simulink model "tqdtqr_rebuild_V3"  (R2021b)
settings: Solver=VariableStepAuto  StartTime=0.0  StopTime=10.0  RelTol=1e-3
undefined symbols (not defined in the file): ATQD_AfterTqMinGain_X_Deg, ATQD_APSCreepBaseTqD_X_kph, ATQD_APSCreepBaseTqD_Y_Deg, ATQD_APSCreepBaseTqR_X_kph, ATQD_APSCreepBaseTqR_Y_Deg, ATQD_APSCreepIterm_X_kph, ATQD_APSCreepIterm_Y_kph, ATQD_APSCreepPterm_X_kph, ATQD_APSCreepPterm_Y_kph, ATQD_APSDecReq_X_kph, ATQD_APSDecReq_Y_mps2, ATQD_APSDecReqCMD_X_kph, ATQD_APSDecReqTs_X_pct, ATQD_APSDecTimeGain_X_Deg, ATQD_APSDecTimeGain_Y_s, ATQD_APSReqLowSpd_X_Deg, ATQD_AutoHoldReleaseBPS_X_Deg, ATQD_AWDLoadTrqnsGain_X_kg, ATQD_AWDLoadTrqnsGain_Y_pct, ATQD_BOSEnBPSPosn_X_kph, ATQD_BOSMap_X_rpm, ATQD_BOSMap_Y_pct, ATQD_CreepBaseTqD_X_kph, ATQD_CreepBaseTqD_Y_Deg, ATQD_CreepBaseTqR_X_kph, ATQD_CreepBaseTqR_Y_Deg, ATQD_CreepBPSDisPosn_X_Deg, ATQD_CreepBPSDisPosnR_X_Deg, ATQD_CreepBPSEnPosn_X_Deg, ATQD_CreepBPSEnPosnR_X_Deg, ATQD_CreepDeltaTq_X_kph, ATQD_CreepIterm_X_kph, ATQD_CreepIterm_Y_kph, ATQD_CreepItermMaxLimit_X_pct, ATQD_CreepPreloadTime_X_kph, ATQD_CreepPreloadTq_X_kph, ATQD_CreepPreloadTq_Y_s, ATQD_CreepProtTq_X_Deg, ATQD_CreepPterm_X_kph, ATQD_CreepPterm_Y_kph, ATQD_CreepRrTqSpRat_X_rpm, ATQD_CreepRrTqSpRat_Y_Nm, ATQD_CreepTargetSpdD_X_pct, ATQD_CreepTargetSpdR_X_pct, ATQD_CreepUpLimitTq_X_rpm, ATQD_DecIneOPDHoldEnDelay_X_Deg, ATQD_DecIneOPDHoldEnDelay_Y_bar, ATQD_ECOTqMapD_X_rpm, ATQD_ECOTqMapD_Y_pct, ATQD_EMTqMapD_X_rpm, ATQD_EMTqMapD_Y_pct, ATQD_EOPDTqMapDCon_X_rpm, ATQD_EOPDTqMapDCon_Y_Deg, ATQD_EstInitVehWeight_X_c, ATQD_FAfterTqCMDGain_X_rpm, ATQD_FAfterTqCMDGain_Y_pct, ATQD_ForceLowSpd_X_Deg, ATQD_ForcePLimitSpd_X_Deg, ATQD_FrLossMAPLowV_X_rpm, ATQD_FrLossMAPLowV_Y_Nm ... (+949)
libraries: simulink x235, hcu_lib x208, tqr x63, tqd x6
(part 22 of 37)

== system tqdtqr_rebuild_V3/Input_Convert/Signal function/OPD Hold/OPDHold Request  ==
  VTQD_VehActSpd_kph : Inport
  VTQD_APSStaSys_enum : Inport  Port=2
  VTQD_AutiHoldRelease_flg : Inport  Port=3
  task_time_s : Inport  Port=4
  VVMC_EstSlope_Deg : Inport  Port=5
  VTQD_OPDHoldForceEn_flg : Inport  Port=6
  AND : Logic  AllPortsSameDT=off  OutDataTypeStr=boolean
  AND1 : Logic  Inputs=3  AllPortsSameDT=off  OutDataTypeStr=boolean
  AND2 : Logic  Operator=OR  AllPortsSameDT=off  OutDataTypeStr=boolean
  AND3 : Logic  AllPortsSameDT=off  OutDataTypeStr=boolean
  AND4 : Logic  AllPortsSameDT=off  OutDataTypeStr=boolean
  Constant1 : Constant  Value=KTQD_APSReqUpSpd_kph
  Constant10 : Constant  Value=KTQD_APSReqDownSpd_kph
  Constant11 : Constant  Value=KTQD_OPDHoldLampDelayTime_s
  Constant12 : Constant  Value=KTQD_OPDHoldLampEnSpd_kph  OutDataTypeStr=single
  Constant13 : Constant  Value=KTQD_OPDHoldLampDisSpd_kph  OutDataTypeStr=single
  Constant14 : Constant  Value=KTQD_ForceAPSReqUpSpd_kph
  Constant15 : Constant  Value=KTQD_APSReqDelayTime_s
  Constant16 : Constant  Value=KTQD_OPDHoldAlarm_flg_ovrdflg
  Constant17 : Constant  Value=KTQD_OPDHoldAlarm_flg_ovrdval
  Constant2 : Constant  Value=2  OutDataTypeStr=uint8
  Constant3 : Constant  Value=2  OutDataTypeStr=uint8
  Constant4 : Constant  OutDataTypeStr=uint8
  Constant5 : Constant  Value=2  OutDataTypeStr=uint8
  Constant6 : Constant  Value=0  OutDataTypeStr=uint8
  Constant7 : Constant  OutDataTypeStr=uint8
  Constant8 : Constant  OutDataTypeStr=uint8
  Constant9 : Constant  Value=KTQD_APSReqDelayTime_s
  Equal1 : RelationalOperator  Operator=<  OutDataTypeStr=boolean  RndMeth=Simplest
  Equal2 : RelationalOperator  Operator=~=  OutDataTypeStr=boolean  RndMeth=Simplest
  Equal3 : RelationalOperator  Operator===  OutDataTypeStr=boolean  RndMeth=Simplest
  Equal4 : RelationalOperator  Operator===  OutDataTypeStr=boolean  RndMeth=Simplest
  Equal5 : RelationalOperator  Operator===  OutDataTypeStr=boolean  RndMeth=Simplest
  Equal6 : RelationalOperator  Operator=>  OutDataTypeStr=boolean  RndMeth=Simplest
  MTQD_APSReqLowSpd_Y_kph : Lookup_n-D  NumberOfTableDimensions=1  BreakpointsForDimension1=ATQD_APSReqLowSpd_X_Deg  Table=MTQD_APSReqLowSpd_Y_kph  InternalRulePriority=Speed  RndMeth=Simplest  InputSameDT=on
  MTQD_ForceLowSpd_Y_kph : Lookup_n-D  NumberOfTableDimensions=1  BreakpointsForDimension1=ATQD_ForceLowSpd_X_Deg  Table=MTQD_ForceLowSpd_Y_kph  InternalRulePriority=Speed  RndMeth=Simplest  InputSameDT=on
  NOT1 : Logic  Operator=NOT  AllPortsSameDT=off  OutDataTypeStr=boolean
  NOT2 : Logic  Operator=NOT  AllPortsSameDT=off  OutDataTypeStr=boolean
  Relational Operator1 : RelationalOperator  Operator=<  OutDataTypeStr=boolean  RndMeth=Simplest
  Relational Operator2 : RelationalOperator  OutDataTypeStr=boolean  RndMeth=Simplest
  Relational Operator3 : RelationalOperator  Operator=<  OutDataTypeStr=boolean  RndMeth=Simplest
  Relational Operator4 : RelationalOperator  Operator=>  OutDataTypeStr=boolean  RndMeth=Simplest
  Relational Operator5 : RelationalOperator  OutDataTypeStr=boolean  RndMeth=Simplest
  Relay : Relay  OnSwitchValue=KTQD_OPDHoldGradeUp_Deg  OffSwitchValue=KTQD_OPDHoldGradeDown_Deg  OutDataTypeStr=boolean
      settings: AttributesFormatString=|
      | On: %<OffSwitchValue>
      | Off: %<OnSwitchValue>
  SR_Latch : hcu_lib/Basic_Blocks/SR_Latch
  SR_Latch1 : hcu_lib/Basic_Blocks/SR_Latch
  Switch{,1..5} (6 alike) : Switch  Criteria=u2 ~= 0
      settings: AttributesFormatString=%<Criteria>
  Timer : hcu_lib/Basic_Blocks/Timer
  VTQD_APSReqTimer_s : Outport
  VTQD_APSReq_enum : Outport  Port=2
  VTQD_APSDecReqA_flg : Outport  Port=3
  VTQD_OPDHoldLamp_flg : Outport  Port=4
  VTQD_OPDHoldAlarm_flg : Outport  Port=5
  wires:
  AND3/1 -> [VTQD_OPDHoldLamp_flg]  "VTQD_OPDHoldLamp_flg"
  SR_Latch1/1 -> AND3/2  "VTQD_OPDHoldSpdEnLamp_flg"
  Equal6/1 -> AND3/1
  Relational Operator4/1 -> SR_Latch1/2
  Constant13/1 -> Relational Operator4/2
  [VTQD_VehActSpd_kph] -> Relational Operator4/1
  Constant12/1 -> Relational Operator3/2
  Relational Operator3/1 -> SR_Latch1/1
  [VTQD_VehActSpd_kph] -> Relational Operator3/1
  [VTQD_OPDHoldLamp_flg] -> VTQD_OPDHoldLamp_flg/1
  [VTQD_APSReqTimer_s] -> Equal6/1
  Constant11/1 -> Equal6/2
  Constant10/1 -> Switch/3
  Constant1/1 -> Switch/1
  Relay/1 -> Switch/2  "VTQD_OPDHoldUpDown_flg"
  [VVMC_EstSlope_Deg] -> Relay/1
  Equal2/1 -> AND2/2
  [VTQD_APSStaSys_enum] -> Equal2/1
  Constant3/1 -> Equal2/2
  [VTQD_AutiHoldRelease_flg] -> AND2/1
  AND2/1 -> SR_Latch/2
  Relational Operator1/1 -> SR_Latch/1
  SR_Latch/1 -> AND1/1
  [VVMC_EstSlope_Deg] -> MTQD_APSReqLowSpd_Y_kph/1
  VVMC_EstSlope_Deg/1 -> [VVMC_EstSlope_Deg]
  [VTQD_AutiHoldRelease_flg] -> NOT1/1
  [VTQD_APSDecReqA_flg] -> VTQD_APSDecReqA_flg/1
  [VTQD_APSReq_enum] -> VTQD_APSReq_enum/1
  [VTQD_APSReqTimer_s] -> VTQD_APSReqTimer_s/1
  task_time_s/1 -> [task_time_s]
  VTQD_AutiHoldRelease_flg/1 -> [VTQD_AutiHoldRelease_flg]
  VTQD_APSStaSys_enum/1 -> [VTQD_APSStaSys_enum]
  VTQD_VehActSpd_kph/1 -> [VTQD_VehActSpd_kph]
  Constant5/1 -> Equal4/2
  AND1/1 -> Timer/1, NOT2/1  "VTQD_APSStasysLow_flg"
  [VTQD_VehActSpd_kph] -> Relational Operator1/1
  [VTQD_APSStaSys_enum] -> Equal4/1
  Equal1/1 -> AND/1
  Switch1/1 -> Switch2/3
  Constant2/1 -> Equal3/2
  [VTQD_APSReq_enum] -> Equal5/1
  Constant7/1 -> Equal5/2
  NOT1/1 -> AND1/3
  [VTQD_APSReqUpSpd_kph] -> Equal1/2
  Equal5/1 -> [VTQD_APSDecReqA_flg]  "VTQD_APSDecReqA_flg"
  [VTQD_VehActSpd_kph] -> Equal1/1
  [VTQD_APSStaSys_enum] -> Equal3/1
  Equal4/1 -> AND1/2
  Constant8/1 -> Switch2/1
  Relational Operator2/1 -> Switch2/2
  Timer/1 -> Relational Operator2/1, [VTQD_APSReqTimer_s]  "VTQD_APSReqTimer_s"
  Constant6/1 -> Switch1/3
  Equal3/1 -> AND/2
  Constant9/1 -> Timer/4, Relational Operator2/2
  AND/1 -> Switch1/2  "VTQD_APSStasysUp_flg"
  Switch2/1 -> [VTQD_APSReq_enum]  "VTQD_APSReq_enum"
  NOT2/1 -> Timer/2
  Constant4/1 -> Switch1/1
  [task_time_s] -> Timer/3
  Constant14/1 -> Switch4/1
  [VTQD_OPDHoldForceEn_flg] -> Switch4/2
  Switch/1 -> Switch4/3
  Switch4/1 -> [VTQD_APSReqUpSpd_kph]  "VTQD_APSReqUpSpd_kph"
  [VVMC_EstSlope_Deg] -> MTQD_ForceLowSpd_Y_kph/1
  MTQD_ForceLowSpd_Y_kph/1 -> Switch3/1  "VTQD_ForceReqLowSpd_kph"
  Switch3/1 -> [VTQD_OPDHoldReqLowSpd_kph]  "VTQD_OPDHoldReqLowSpd_kph"
  [VTQD_OPDHoldForceEn_flg] -> Switch3/2
  MTQD_APSReqLowSpd_Y_kph/1 -> Switch3/3  "VTQD_APSReqLowSpd_kph"
  [VTQD_OPDHoldReqLowSpd_kph] -> Relational Operator1/2
  Constant15/1 -> Relational Operator5/2
  AND4/1 -> Switch5/3
  Constant16/1 -> Switch5/2
  [VTQD_APSReqTimer_s] -> Relational Operator5/1
  Switch5/1 -> [VTQD_OPDHoldAlarm_flg]  "VTQD_OPDHoldAlarm_flg"
  Constant17/1 -> Switch5/1
  Relational Operator5/1 -> AND4/1
  [VTQD_OPDHoldForceEn_flg] -> AND4/2
  VTQD_OPDHoldForceEn_flg/1 -> [VTQD_OPDHoldForceEn_flg]
  [VTQD_OPDHoldAlarm_flg] -> VTQD_OPDHoldAlarm_flg/1

== system tqdtqr_rebuild_V3/Input_Convert/Signal function/OPD Hold/Parking Requeest Backup ==
  note: Park request
  note: Allow park
  VTQD_APSReq_enum : Inport
  VTQD_APSReqTimer_s : Inport  Port=2
  VTQD_ParkRequest_flg : Inport  Port=3
  task_time_s : Inport  Port=4
  VTQD_AutiHoldRelease_flg : Inport  Port=5
  AND : Logic  AllPortsSameDT=off  OutDataTypeStr=boolean
  AND1 : Logic  AllPortsSameDT=off  OutDataTypeStr=boolean
  AND3 : Logic  Inputs=3  AllPortsSameDT=off  OutDataTypeStr=boolean
  Constant1 : Constant  Value=KTQD_APSReqDelayTime_s
  Constant16 : Constant  OutDataTypeStr=uint8
  Constant17 : Constant  Value=TRUE  OutDataTypeStr=uint8
  Constant2 : Constant  Value=KTQD_APSReqDelayTime_s
  Constant3 : Constant  Value=KTQD_OPDHoldBrkSW_flg
  Constant4 : Constant  Value=KTQD_OPDHoldAllowPark_flg
  Constant5 : Constant  Value=KTQD_OPDHoldAllowPark_s
  Constant6 : Constant  Value=KTQD_OPDHoldAllowGearPSW_flg
  DelayEnable : hcu_lib/Basic_Blocks/DelayEnable
  Equal6 : RelationalOperator  Operator===  OutDataTypeStr=boolean  RndMeth=Simplest
  NOT : Logic  Operator=NOT  AllPortsSameDT=off  OutDataTypeStr=boolean
  OR : Logic  Operator=OR  AllPortsSameDT=off  OutDataTypeStr=boolean
  Relational Operator1 : RelationalOperator  OutDataTypeStr=boolean  RndMeth=Simplest
  Relational Operator6 : RelationalOperator  OutDataTypeStr=boolean  RndMeth=Simplest
  SR_Latch : hcu_lib/Basic_Blocks/SR_Latch
  Switch4 : Switch  Criteria=u2 ~= 0
      settings: AttributesFormatString=%<Criteria>
  VTQD_ActParkRequest_flg : Outport
  VTQD_OPDHoldAllowPark_flg : Outport  Port=2
  wires:
  [VTQD_OPDHoldAllowPark_flg] -> VTQD_OPDHoldAllowPark_flg/1
  Constant6/1 -> NOT/1
  NOT/1 -> AND1/2
  AND1/1 -> OR/2
  [VTQD_OPDHoldAllowPark_flg] -> AND1/1
  [task_time_s] -> DelayEnable/3
  AND3/1 -> OR/1
  OR/1 -> Switch4/2
  SR_Latch/1 -> [VTQD_OPDHoldAllowPark_flg]  "VTQD_OPDHoldAllowPark_flg"
  VTQD_AutiHoldRelease_flg/1 -> [VTQD_AutiHoldRelease_flg]
  [VTQD_AutiHoldRelease_flg] -> SR_Latch/2
  DelayEnable/1 -> SR_Latch/1
  Constant5/1 -> DelayEnable/2
  Constant4/1 -> AND/2
  Relational Operator1/1 -> AND/1
  AND/1 -> DelayEnable/1
  task_time_s/1 -> [task_time_s]
  [VTQD_APSReqTimer_s] -> Relational Operator1/1
  Constant2/1 -> Relational Operator1/2
  [VTQD_ActParkRequest_flg] -> VTQD_ActParkRequest_flg/1
  VTQD_ParkRequest_flg/1 -> [VTQD_ParkRequest_flg]
  VTQD_APSReqTimer_s/1 -> [VTQD_APSReqTimer_s]
  VTQD_APSReq_enum/1 -> [VTQD_APSReq_enum]
  [VTQD_APSReqTimer_s] -> Relational Operator6/1
  Switch4/1 -> [VTQD_ActParkRequest_flg]  "VTQD_ActParkRequest_flg"
  Constant16/1 -> Equal6/2
  Constant17/1 -> Switch4/1
  [VTQD_ParkRequest_flg] -> Switch4/3
  Relational Operator6/1 -> AND3/3
  [VTQD_APSReq_enum] -> Equal6/1
  Equal6/1 -> AND3/1
  Constant1/1 -> Relational Operator6/2
  Constant3/1 -> AND3/2

== system tqdtqr_rebuild_V3/Input_Convert/Signal function/OPD Hold/Release Condition ==
  note: Release auto hold
  note: OPD release in reverse condition
  note: OPD Enable Flag
  note: Calculate Tq to release OPD disable
  note: Calulaye Tq to release OPD enable
  note: OPD detect time
  VVMC_EstSlope_Deg : Inport
  VTQD_VehActSpd_kph : Inport  Port=2
  VTQR_NoABSFEDUWhlTqReq_Nm : Inport  Port=3
  VTQR_NoABSREDUWhlTqReq_Nm : Inport  Port=4
  VTQD_ActBPSPosn_pct : Inport  Port=5
  task_time_s : Inport  Port=6
  VTQD_APSReqTimer_s : Inport  Port=7
  VTQD_LowIdleAccPedal_flg : Inport  Port=8
  VTQD_OPDHoldRgnOn2Off_flg : Inport  Port=9
  AND : Logic  Inputs=3  AllPortsSameDT=off  OutDataTypeStr=boolean
  AND1 : Logic  AllPortsSameDT=off  OutDataTypeStr=boolean
  AND2 : Logic  AllPortsSameDT=off  OutDataTypeStr=boolean
  AND3 : Logic  AllPortsSameDT=off  OutDataTypeStr=boolean
  Add : Sum
  Add1 : Sum  Inputs=+-+
  Add6 : Sum
  Add7 : Sum
  Constant1 : Constant  Value=KTQD_APSRelDisTqDev_Nm
  Constant{5,10,23,30} (4 alike) : Constant  Value=ZERO_FLOAT
  Constant2 : Constant  Value=KTQD_OPDHoldDownEnTime_s
  Constant36 : Constant  Value=KTQD_OPDHoldRelDetSpd_kph
  Constant4 : Constant  Value=KTQD_OPDHoldRelTqGain_Nm
  Constant6 : Constant  Value=KTQD_OPDHoldDetRevSpd_kph
  Constant7 : Constant  Value=KTQD_OPDHoldLiftRevSpd_kph
  Constant8 : Constant  Value=KTQD_APSDecReqMaxTime_s
  Constant9 : Constant  Value=KTQD_OPDHoldRelTqGain_Nm
  Delay{,1..2,4..7} (7 alike) : Delay  DelayLength=1  InitialCondition=single(0)
      settings: AttributesFormatString=%<InitialCondition>
  Delay3 : Delay  DelayLength=1
  DelayEnable : hcu_lib/Basic_Blocks/DelayEnable
  DelayEnable1 : hcu_lib/Basic_Blocks/DelayEnable
  Detect Increase : simulink/Logic and Bit Operations/Detect Increase  vinit=0.0  OutDataTypeStr=boolean
  Detect Increase1 : simulink/Logic and Bit Operations/Detect Increase  vinit=0.0  OutDataTypeStr=boolean
  Detect Increase2 : simulink/Logic and Bit Operations/Detect Increase  vinit=0.0  OutDataTypeStr=boolean
  MTQD_AutoHoldReleaseBPS_Y_pct : Lookup_n-D  NumberOfTableDimensions=1  BreakpointsForDimension1=ATQD_AutoHoldReleaseBPS_X_Deg  Table=MTQD_AutoHoldReleaseBPS_Y_pct  InternalRulePriority=Speed  RndMeth=Simplest  InputSameDT=on
  MTQD_OPDHoldDownRelDelay_Y_s : Lookup_n-D  NumberOfTableDimensions=1  BreakpointsForDimension1=ATQD_OPDHoldDownRelDelay_X_Deg  Table=MTQD_OPDHoldDownRelDelay_Y_s  InternalRulePriority=Speed  RndMeth=Simplest  InputSameDT=on
  MTQD_OPDHoldRelDetTime_Y_s : Lookup_n-D  NumberOfTableDimensions=1  BreakpointsForDimension1=ATQD_OPDHoldRelDetTime_X_Deg  Table=MTQD_OPDHoldRelDetTime_Y_s  InternalRulePriority=Speed  RndMeth=Simplest  InputSameDT=on
  MTQD_OPDHoldReleaseTq_Y_Nm{,1..3} (4 alike) : Lookup_n-D  NumberOfTableDimensions=1  BreakpointsForDimension1=ATQD_OPDHoldReleaseTq_X_Deg  Table=MTQD_OPDHoldReleaseTq_Y_Nm  InternalRulePriority=Speed  RndMeth=Simplest  InputSameDT=on
  Max : MinMax  Function=max  Inputs=2
  Max1 : MinMax  Function=max  Inputs=2
  Max2 : MinMax  Function=max  Inputs=2
  NOT{,1..5} (6 alike) : Logic  Operator=NOT  AllPortsSameDT=off  OutDataTypeStr=boolean
  OR : Logic  Operator=OR  AllPortsSameDT=off  OutDataTypeStr=boolean
  OR1 : Logic  Operator=OR  AllPortsSameDT=off  OutDataTypeStr=boolean
  OR2 : Logic  Operator=OR  AllPortsSameDT=off  OutDataTypeStr=boolean
  OR3 : Logic  Operator=OR  Inputs=3  AllPortsSameDT=off  OutDataTypeStr=boolean
  Relational Operator : RelationalOperator  Operator=>  OutDataTypeStr=boolean  RndMeth=Simplest
  Relational Operator1 : RelationalOperator  Operator=<=  OutDataTypeStr=boolean  RndMeth=Simplest
  Relational Operator3 : RelationalOperator  Operator=<=  OutDataTypeStr=boolean  RndMeth=Simplest
  Relational Operator4 : RelationalOperator  OutDataTypeStr=boolean  RndMeth=Simplest
  Relational Operator5 : RelationalOperator  Operator=<  OutDataTypeStr=boolean  RndMeth=Simplest
  Relational Operator6 : RelationalOperator  Operator=>  OutDataTypeStr=boolean  RndMeth=Simplest
  Relational Operator7 : RelationalOperator  OutDataTypeStr=boolean  RndMeth=Simplest
  Relational Operator9 : RelationalOperator  OutDataTypeStr=boolean  RndMeth=Simplest
  Relay : Relay  OnSwitchValue=KTQD_OPDHoldGradeUp_Deg  OffSwitchValue=KTQD_OPDHoldGradeDown_Deg  OutDataTypeStr=boolean
      settings: AttributesFormatString=|
      | Off: %<OffSwitchValue>
      | On: %<OnSwitchValue>
  Relay1 : Relay  OnSwitchValue=KTQD_OPDHoldGradeUp_Deg  OffSwitchValue=KTQD_OPDHoldGradeDown_Deg  OutDataTypeStr=boolean
      settings: AttributesFormatString=|
      | Off: %<OffSwitchValue>
      | On: %<OnSwitchValue>
  SR_Latch : hcu_lib/Basic_Blocks/SR_Latch
  SR_Latch1 : hcu_lib/Basic_Blocks/SR_Latch
  Switch{,1..6} (7 alike) : Switch  Criteria=u2 ~= 0
      settings: AttributesFormatString=%<Criteria>
  VTQD_AutoHoldRelease_flg : Outport
  VTQD_OPDHoldEnRel_flg : Outport  Port=2
  VTQD_OPDHoldActRelTq_Nm : Outport  Port=3
  wires:
  [VTQD_OPDHoldActRelTq_Nm] -> VTQD_OPDHoldActRelTq_Nm/1
  OR3/1 -> SR_Latch1/2
  [VVMC_EstSlope_Deg] -> MTQD_OPDHoldReleaseTq_Y_Nm2/1
  Max/1 -> Switch4/1
  Relational Operator6/1 -> OR3/2
  NOT1/1 -> OR1/2
  Constant1/1 -> Add1/2
  [VTQD_OPDHoldEnRel_flg] -> AND2/1
  [VTQD_VehActSpd_kph] -> Relational Operator6/1
  NOT2/1 -> AND1/1
  Switch/1 -> OR/2
  Constant9/1 -> Switch3/1
  AND3/1 -> OR3/3
  Constant5/1 -> Switch2/3
  Switch4/1 -> Add1/3, Delay2/1
  Constant7/1 -> Relational Operator6/2
  Relational Operator7/1 -> AND3/2
  Delay1/1 -> Relational Operator7/1
  MTQD_OPDHoldReleaseTq_Y_Nm3/1 -> Max2/2
  [VVMC_EstSlope_Deg] -> MTQD_OPDHoldReleaseTq_Y_Nm1/1
  Switch3/1 -> Add1/1
  [VTQD_OPDHoldRelReverse_flg] -> Switch2/2
  Add6/1 -> Relational Operator4/1  "VTQD_OPDHoldEnRelTq_Nm"
  [VTQD_LowIdleAccPedal_flg] -> Detect Increase/1
  MTQD_OPDHoldReleaseTq_Y_Nm2/1 -> Max/2
  Constant10/1 -> Switch3/3
  [VTQD_APSReqTimer_s] -> Delay1/1
  NOT4/1 -> DelayEnable1/1
  Constant36/1 -> Relational Operator9/2
  [VTQD_LowIdleAccPedal_flg] -> NOT5/1
  [VTQD_LowIdleAccPedal_flg] -> AND3/1
  AND1/1 -> Switch/1
  [VTQD_OPDHoldEnRel_flg] -> AND1/2
  Delay2/1 -> Max/1
  [VTQD_VehActSpd_kph] -> Relational Operator3/1
  OR2/1 -> SR_Latch/2
  Constant8/1 -> Relational Operator7/2
  Delay/1 -> Relational Operator1/1
  [VTQD_OPDHoldRelReverse_flg] -> Switch4/2
  Add/1 -> [VTQD_OPDHoldActRelTq_Nm]  "VTQD_OPDHoldActRelTq_Nm"
  Relay/1 -> NOT/1
  MTQD_OPDHoldReleaseTq_Y_Nm1/1 -> Switch4/3
  NOT5/1 -> AND2/2
  Switch2/1 -> Add/1
  [VTQD_OPDHoldRelReverse_flg] -> Switch3/2
  MTQD_OPDHoldRelDetTime_Y_s/1 -> Switch5/3
  [VTQD_LowIdleAccPedal_flg] -> NOT4/1
  Constant23/1 -> Max1/2
  [VTQD_OPDHoldRelReverse_flg] -> Switch6/2
  [VTQD_OPDHoldRelReverse_flg] -> Detect Increase2/1
  NOT3/1 -> Switch1/2
  [VTQD_APSReqTimer_s] -> Delay/1
  [VVMC_EstSlope_Deg] -> MTQD_OPDHoldReleaseTq_Y_Nm3/1
  Switch6/1 -> Delay3/1, Add/2  "VTQD_OPDHoldReleaseTq_Nm"
  Add7/1 -> Relational Operator5/1  "VTQD_OPDHoldDisRelTq_Nm"
  Detect Increase/1 -> OR3/1
  Constant6/1 -> Relational Operator3/2
  Max2/1 -> Switch6/1
  Delay3/1 -> Max2/1
  [VTQD_OPDHoldDownRelDelay_s] -> DelayEnable1/2
  Relational Operator3/1 -> Detect Increase1/1
  MTQD_OPDHoldReleaseTq_Y_Nm/1 -> Switch6/3
  OR/1 -> [VTQD_AutoHoldRelease_flg]  "VTQD_AutoHoldRelease_flg"
  MTQD_AutoHoldReleaseBPS_Y_pct/1 -> Relational Operator/2  "VTQD_AutoHoldReleaseAPS_pct"
  Switch5/1 -> [VTQD_OPDHoldRelDetTime_s]  "VTQD_OPDHoldRelDetTime_s"
  [VVMC_EstSlope_Deg] -> MTQD_OPDHoldRelDetTime_Y_s/1
  [VVMC_EstSlope_Deg] -> MTQD_AutoHoldReleaseBPS_Y_pct/1
  Relational Operator9/1 -> Switch5/2
  [VTQD_VehActSpd_kph] -> Relational Operator9/1
  Max1/1 -> Relational Operator5/2
  [VTQR_NoABSREDUWhlTqReq_Nm] -> Delay7/1
  DelayEnable/1 -> [VTQD_OPDHoldEnRel_flg]  "VTQD_OPDHoldEnRel_flg"
  [VVMC_EstSlope_Deg] -> MTQD_OPDHoldReleaseTq_Y_Nm/1
  Add1/1 -> Max1/1
  [VTQD_ActBPSPosn_pct] -> Relational Operator/1
  [task_time_s] -> DelayEnable/3
  [VTQR_NoABSREDUWhlTqReq_Nm] -> Delay5/1
  [VTQR_NoABSFEDUWhlTqReq_Nm] -> Delay4/1
  [VVMC_EstSlope_Deg] -> Relay/1
  AND/1 -> OR/1
  [VTQD_OPDHoldRelDetTime_s] -> DelayEnable/2
  Relational Operator1/1 -> AND/1
  Relational Operator/1 -> OR1/1
  [VTQD_OPDHoldRgnOn2Off_flg] -> Switch/2
  [VTQD_LowIdleAccPedal_flg] -> NOT1/1
  AND2/1 -> Switch1/3
  Switch1/1 -> Switch/3
  OR1/1 -> AND/3
  Constant2/1 -> Relational Operator1/2
  Relay1/1 -> NOT3/1
  [VVMC_EstSlope_Deg] -> Relay1/1
  NOT/1 -> AND/2
  Constant30/1 -> Switch5/1
  [VTQD_LowIdleAccPedal_flg] -> NOT2/1
  [task_time_s] -> DelayEnable1/3
  [VVMC_EstSlope_Deg] -> MTQD_OPDHoldDownRelDelay_Y_s/1
  Constant4/1 -> Switch2/1
  MTQD_OPDHoldDownRelDelay_Y_s/1 -> [VTQD_OPDHoldDownRelDelay_s]  "VTQD_OPDHoldDownRelDelay_s"
  SR_Latch1/1 -> [VTQD_OPDHoldRelReverse_flg]  "VTQD_OPDHoldRelReverse_flg"
  DelayEnable1/1 -> Switch1/1
  Detect Increase1/1 -> SR_Latch1/1
  Detect Increase2/1 -> OR2/1
  SR_Latch/1 -> DelayEnable/1  "VTQD_OPDHoldEnRelLatch_flg"
  VTQD_OPDHoldRgnOn2Off_flg/1 -> [VTQD_OPDHoldRgnOn2Off_flg]
  VTQD_LowIdleAccPedal_flg/1 -> [VTQD_LowIdleAccPedal_flg]
  VTQD_APSReqTimer_s/1 -> [VTQD_APSReqTimer_s]
  [VTQD_OPDHoldEnRel_flg] -> VTQD_OPDHoldEnRel_flg/1
  [VTQD_AutoHoldRelease_flg] -> VTQD_AutoHoldRelease_flg/1
  task_time_s/1 -> [task_time_s]
  VTQD_ActBPSPosn_pct/1 -> [VTQD_ActBPSPosn_pct]
  VTQR_NoABSREDUWhlTqReq_Nm/1 -> [VTQR_NoABSREDUWhlTqReq_Nm]
  VTQR_NoABSFEDUWhlTqReq_Nm/1 -> [VTQR_NoABSFEDUWhlTqReq_Nm]
  VTQD_VehActSpd_kph/1 -> [VTQD_VehActSpd_kph]
  VVMC_EstSlope_Deg/1 -> [VVMC_EstSlope_Deg]
  Relational Operator4/1 -> [VTQD_OPDHoldEnRelease_flg]  "VTQD_OPDHoldEnRelease_flg"
  [VTQD_OPDHoldEnRelease_flg] -> SR_Latch/1
  [VTQD_OPDHoldActRelTq_Nm] -> Relational Operator4/2
  Relational Operator5/1 -> [VTQD_OPDHoldDisRelease_flg]  "VTQD_OPDHoldDisRelease_flg"
  [VTQD_OPDHoldDisRelease_flg] -> OR2/2
  Delay4/1 -> Add6/1
  Delay5/1 -> Add6/2
  Delay6/1 -> Add7/1
  [VTQR_NoABSFEDUWhlTqReq_Nm] -> Delay6/1
  Delay7/1 -> Add7/2

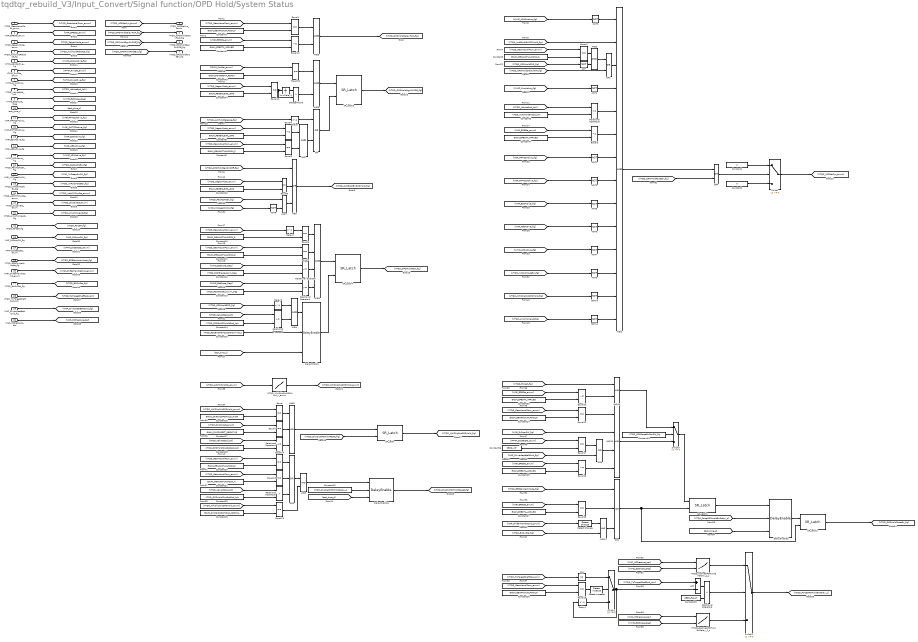
== system tqdtqr_rebuild_V3/Input_Convert/Signal function/OPD Hold/System Status ==
  VTQD_GearActualPosn_enum : Inport
  VINP_EPBSta_enum : Inport  Port=2
  VTQD_RegenMode_enum : Inport  Port=3
  VTQD_AutiHoldRelease_flg : Inport  Port=4
  VVMC_ADASActive_flg : Inport  Port=5
  VPMM_PwrSta_enum : Inport  Port=6
  VVMC_CruzActive_flg : Inport  Port=7
  VTQD_VehActSpd_kph : Inport  Port=8
  VVMC_EstSlope_Deg : Inport  Port=9
  task_time_s : Inport  Port=10
  VINP_FrPTCSActive_flg : Inport  Port=11
  VINP_RrPTCSActive_flg : Inport  Port=12
  VINP_ESCActive_flg : Inport  Port=13
  VINP_ABSActive_flg : Inport  Port=14
  VVMC_APSActive_flg : Inport  Port=15
  VTQD_PedAccTqEn_flg : Inport  Port=16
  VINP_IVICreepOnSW_flg : Inport  Port=17
  VTQD_IVIRockModeEn_flg : Inport  Port=18
  VTQD_ActWhlSkipSta_enum : Inport  Port=19
  VTQD_SkipDirect_enum : Inport  Port=20
  VTQD_LimpHomeAct_flg : Inport  Port=21
  VTQD_ForceP_flg : Inport  Port=22
  VINP_DrDoorSW_flg : Inport  Port=23
  VPMM_DrSeatSta_enum : Inport  Port=24
  VTQD_EPBCarWashMode_flg : Inport  Port=25
  VINP_ShifterHandleCmd_enum : Inport  Port=26
  VTQD_BrkSwSta_flg : Inport  Port=27
  VTQD_TqTargetShaftSpd_rpm : Inport  Port=28
  VINP_DriverSeatBeltCmd_flg : Inport  Port=29
  VINP_MCPressure_bar : Inport  Port=30
  AND{,3..7,9..11} (9 alike) : Logic  AllPortsSameDT=off  OutDataTypeStr=boolean
  AND1 : Logic  Inputs=4  AllPortsSameDT=off  OutDataTypeStr=boolean
  AND12 : Logic  Inputs=4  AllPortsSameDT=off  OutDataTypeStr=boolean
  AND2 : Logic  Inputs=14  AllPortsSameDT=off  OutDataTypeStr=boolean
  AND8 : Logic  Inputs=3  AllPortsSameDT=off  OutDataTypeStr=boolean
  Abs : Abs
  Add : Sum  Inputs=+-
  Constant1 : Constant  Value=2  OutDataTypeStr=uint8
  Constant10 : Constant  Value=ENUM_GEARACTUALPOSN_R
  Constant11 : Constant  Value=ENUM_GEARACTUALPOSN_D
  Constant12 : Constant  Value=KTQD_R2DGradeUpLim_Deg
  Constant13 : Constant  Value=KTQD_R2DGradeLowLim_Deg
  Constant14 : Constant  Value=KTQD_R2DEnOPDHoldSpd_kph
  Constant15 : Constant  Value=KTQD_R2DEnOPDHSpdDelayTime_s
  Constant16 : Constant  Value=ENUM_SKIPDISOPDHOLD_HIGH
  Constant17 : Constant  Value=ENUM_SKIPDIRECT_NEGATIVE
  Constant18 : Constant  Value=KTQD_OPDHoldSkipDetSpd_kph
  Constant19 : Constant  Value=ENUM_SKIPDISOPDHOLD_NORMAL
  Constant2 : Constant  Value=0  OutDataTypeStr=uint8
  Constant{4,9,20,24,28} (5 alike) : Constant  Value=ENUM_GEARACTUALPOSN_P
  Constant21 : Constant  Value=ENUM_GEARACTUALPOSN_N
  Constant22 : Constant  Value=KTQD_SkipRecOPDHoldDelay_s
  Constant23 : Constant  Value=KTQD_OPDHoldSkipDetSpd_kph
  Constant{3,7,25,27,30} (5 alike) : Constant  Value=ENUM_EPBSTA_APPLIED
  Constant26 : Constant  Value=ZERO_INT
  Constant29 : Constant  Value=ZERO_FLOAT
  Constant31 : Constant  Value=KTQD_OPDForceEnConSW_flg
  Constant40 : Constant  Value=ENUM_REGENLEVEL_OPD
  Constant44 : Constant  Value=ENUM_REGENLEVEL_OPD
  Constant45 : Constant  Value=ENUM_POWERSTA_READY
  Constant5 : Constant  Value=ENUM_GEARACTUALPOSN_D
  Constant6 : Constant  Value=KTQD_AutoHoldEnSpd_kph
  Constant8 : Constant  Value=ENUM_REGENLEVEL_OPD
  Delay : Delay  DelayLength=1  InitialCondition=boolean(0)
      settings: AttributesFormatString=%<InitialCondition>
  Delay1 : Delay  DelayLength=1  InitialCondition=single(0)
      settings: AttributesFormatString=%<InitialCondition>
  Delay2 : Delay  DelayLength=1  InitialCondition=uint8(0)
      settings: AttributesFormatString=%<InitialCondition>
  Delay3 : Delay  DelayLength=1  InitialCondition=boolean(0)
      settings: AttributesFormatString=%<InitialCondition>
  DelayEnable : hcu_lib/Basic_Blocks/DelayEnable
  DelayEnable1 : hcu_lib/Basic_Blocks/DelayEnable
  DelayEnable2 : hcu_lib/Basic_Blocks/DelayEnable
  Detect Change : simulink/Logic and Bit Operations/Detect Change  vinit=boolean(0)  OutDataTypeStr=boolean
  Detect Increase : simulink/Logic and Bit Operations/Detect Increase  vinit=boolean(0)  OutDataTypeStr=boolean
  Equal{,1..2,5..9,11..15,17..19,30} (17 alike) : RelationalOperator  Operator===  OutDataTypeStr=boolean  RndMeth=Simplest
  Equal{3..4,10,16,20} (5 alike) : RelationalOperator  Operator=~=  OutDataTypeStr=boolean  RndMeth=Simplest
  GreaterThan3 : RelationalOperator  Operator=>  OutDataTypeStr=boolean  RndMeth=Simplest
  MTQD_AccIneOPDHoldEnDelay_Z_s : Lookup_n-D  BreakpointsForDimension1=ATQD_DecIneOPDHoldEnDelay_Y_bar  BreakpointsForDimension2=ATQD_DecIneOPDHoldEnDelay_X_Deg  Table=MTQD_AccIneOPDHoldEnDelay_Z_s  ExtrapMethod=Clip  InternalRulePriority=Speed  RndMeth=Simplest  InputSameDT=on
      settings: InputPortMap=u0,u1
  MTQD_DecIneOPDHoldEnDelay_Z_s : Lookup_n-D  BreakpointsForDimension1=ATQD_DecIneOPDHoldEnDelay_Y_bar  BreakpointsForDimension2=ATQD_DecIneOPDHoldEnDelay_X_Deg  Table=MTQD_DecIneOPDHoldEnDelay_Z_s  ExtrapMethod=Clip  InternalRulePriority=Speed  RndMeth=Simplest  InputSameDT=on
      settings: InputPortMap=u0,u1
  MTQD_WhlSkipDisOPDHold_Y_enum : Lookup_n-D  NumberOfTableDimensions=1  BreakpointsForDimension1=ATQD_WhlSkipDisOPDHold_X_enum  BreakpointsForDimension1DataTypeStr=uint8  Table=MTQD_WhlSkipDisOPDHold_Y_enum  TableDataTypeStr=uint8  IntermediateResultsDataTypeStr=uint8  ExtrapMethod=Clip  UseLastTableValue=on  InternalRulePriority=Speed  OutDataTypeStr=uint8  RndMeth=Simplest  InputSameDT=on
  NOT{,1..11} (12 alike) : Logic  Operator=NOT  AllPortsSameDT=off  OutDataTypeStr=boolean
  OR{,1,4,6} (4 alike) : Logic  Operator=OR  AllPortsSameDT=off  OutDataTypeStr=boolean
  OR2 : Logic  Operator=OR  Inputs=3  AllPortsSameDT=off  OutDataTypeStr=boolean
  OR3 : Logic  Operator=OR  Inputs=3  AllPortsSameDT=off  OutDataTypeStr=boolean
  OR5 : Logic  Operator=OR  Inputs=3  AllPortsSameDT=off  OutDataTypeStr=boolean
  Relational Operator : RelationalOperator  Operator=<=  OutDataTypeStr=boolean  RndMeth=Simplest
  Relational Operator1 : RelationalOperator  OutDataTypeStr=boolean  RndMeth=Simplest
  Relational Operator2 : RelationalOperator  OutDataTypeStr=boolean  RndMeth=Simplest
  Relational Operator3 : RelationalOperator  Operator=<=  OutDataTypeStr=boolean  RndMeth=Simplest
  Relational Operator4 : RelationalOperator  Operator=<=  OutDataTypeStr=boolean  RndMeth=Simplest
  Relational Operator5 : RelationalOperator  Operator=>  OutDataTypeStr=boolean  RndMeth=Simplest
  Relational Operator6 : RelationalOperator  Operator=<  OutDataTypeStr=boolean  RndMeth=Simplest
  SR_Latch{,1..4} (5 alike) : hcu_lib/Basic_Blocks/SR_Latch
  Switch{,1..3} (4 alike) : Switch  Criteria=u2 ~= 0
      settings: AttributesFormatString=%<Criteria>
  Unit Delay1 : UnitDelay  InitialCondition=boolean(0)  SampleTime=-1  HasFrameUpgradeWarning=on
      settings: AttributesFormatString=%<InitialCondition>
  VTQD_APSStaSys_enum : Outport
  VTQD_OPDHoldDelayForP_flg : Outport  Port=2
  VTQD_OPDHoldRgnOn2Off_flg : Outport  Port=3
  VTQD_OPDHoldForceEn_flg : Outport  Port=4
  wires:
  VTQD_LimpHomeAct_flg/1 -> [VTQD_LimpHomeAct_flg]
  NOT11/1 -> AND2/14
  [VTQD_LimpHomeAct_flg] -> NOT11/1
  NOT10/1 -> AND2/13
  [VTQD_WhlSkipDisOPDHold_flg] -> NOT10/1
  SR_Latch/1 -> [VTQD_WhlSkipDisOPDHold_flg]  "VTQD_WhlSkipDisOPDHold_flg"
  [VTQD_SkipDisOPDHoldReset_flg] -> SR_Latch/2
  DelayEnable1/1 -> [VTQD_SkipDisOPDHoldReset_flg]  "VTQD_SkipDisOPDHoldReset_flg"
  AND9/1 -> DelayEnable1/1
  Equal13/1 -> AND9/2
  OR3/1 -> AND9/1
  Relational Operator5/1 -> OR3/3
  [VTQD_VehActSpd_kph] -> Relational Operator5/1
  Constant23/1 -> Relational Operator5/2
  Constant18/1 -> Relational Operator4/2
  [VTQD_VehActSpd_kph] -> Relational Operator4/1
  Relational Operator4/1 -> AND8/3
  Constant22/1 -> DelayEnable1/2
  [task_time_s] -> DelayEnable1/3
  Equal15/1 -> OR3/2
  Equal14/1 -> OR3/1
  Constant20/1 -> Equal14/2
  Constant21/1 -> Equal15/2
  [VTQD_GearActualPosn_enum] -> Equal15/1
  [VTQD_GearActualPosn_enum] -> Equal14/1
  [VTQD_WhlSkipDisOPDHold_enum] -> Equal13/1
  Constant19/1 -> Equal13/2
  AND8/1 -> SR_Latch/1
  Equal7/1 -> AND8/2
  Equal/1 -> AND8/1
  [VTQD_SkipDirect_enum] -> Equal7/1
  Constant17/1 -> Equal7/2
  Constant16/1 -> Equal/2
  [VTQD_WhlSkipDisOPDHold_enum] -> Equal/1
  MTQD_WhlSkipDisOPDHold_Y_enum/1 -> [VTQD_WhlSkipDisOPDHold_enum]  "VTQD_WhlSkipDisOPDHold_enum"
  [VTQD_ActWhlSkipSta_enum] -> MTQD_WhlSkipDisOPDHold_Y_enum/1
  VTQD_ActWhlSkipSta_enum/1 -> [VTQD_ActWhlSkipSta_enum]
  VTQD_SkipDirect_enum/1 -> [VTQD_SkipDirect_enum]
  NOT1/1 -> AND2/7
  NOT2/1 -> AND2/8
  NOT9/1 -> AND2/12
  [VTQD_IVIRockModeEn_flg] -> NOT9/1
  VTQD_IVIRockModeEn_flg/1 -> [VTQD_IVIRockModeEn_flg]
  VTQD_PedAccTqEn_flg/1 -> [VTQD_PedAccTqEn_flg]
  VINP_IVICreepOnSW_flg/1 -> [VINP_IVICreepOnSW_flg]
  [VTQD_PedAccTqEn_flg] -> AND7/1
  Equal8/1 -> OR5/2
  OR5/1 -> [VTQD_AntiBlockEnOPDHold_flg]  "VTQD_AntiBlockEnOPDHold_flg"
  AND7/1 -> OR5/3
  [VTQD_RegenMode_enum] -> Equal8/1
  [VTQD_OPDHoldRgnOn2Off_flg] -> OR5/1
  Constant40/1 -> Equal8/2
  [VINP_IVICreepOnSW_flg] -> NOT8/1
  NOT8/1 -> AND7/2
  VVMC_APSActive_flg/1 -> [VVMC_APSActive_flg]
  [VVMC_APSActive_flg] -> NOT7/1
  NOT7/1 -> AND2/11
  VINP_RrPTCSActive_flg/1 -> [VINP_RrPTCSActive_flg]
  VINP_ESCActive_flg/1 -> [VINP_ESCActive_flg]
  VINP_FrPTCSActive_flg/1 -> [VINP_FrPTCSActive_flg]
  VINP_ABSActive_flg/1 -> [VINP_ABSActive_flg]
  task_time_s/1 -> [task_time_s]
  VVMC_EstSlope_Deg/1 -> [VVMC_EstSlope_Deg]
  [VINP_FrPTCSActive_flg] -> NOT1/1
  [VVMC_ADASActive_flg] -> NOT3/1
  [VTQD_OPDHoldDelayForP_flg] -> OR1/2
  [VTQD_AntiBlockEnOPDHold_flg] -> AND2/2
  Constant5/1 -> Equal2/2
  [VTQD_OPDHoldR2D_flg] -> NOT/1
  NOT/1 -> AND3/2
  [VTQD_GearActualPosn_enum] -> Equal2/1
  Equal2/1 -> AND3/1
  AND3/1 -> OR1/1
  [VVMC_CruzActive_flg] -> NOT4/1
  [VINP_RrPTCSActive_flg] -> NOT2/1
  NOT5/1 -> AND2/9
  Constant7/1 -> Equal3/2
  [VINP_EPBSta_enum] -> Equal3/1
  [VINP_ESCActive_flg] -> NOT5/1
  NOT6/1 -> AND2/10
  [VINP_ABSActive_flg] -> NOT6/1
  NOT4/1 -> AND2/4
  NOT3/1 -> AND2/1
  Equal3/1 -> AND2/6
  Constant6/1 -> Relational Operator3/2
  OR1/1 -> AND2/3
  Relational Operator3/1 -> AND2/5
  [VTQD_VehActSpd_kph] -> Relational Operator3/1
  Relational Operator2/1 -> AND4/2
  Equal9/1 -> AND1/2
  SR_Latch4/1 -> [VTQD_OPDHoldR2D_flg]  "VTQD_OPDHoldR2D_flg"
  Equal6/1 -> AND1/1
  [VVMC_EstSlope_Deg] -> Relational Operator/1
  Delay3/1 -> AND4/1
  Constant15/1 -> DelayEnable/2
  Relational Operator/1 -> AND1/3
  AND1/1 -> SR_Latch4/1
  Relational Operator1/1 -> AND1/4
  Constant10/1 -> Equal6/2
  AND4/1 -> DelayEnable/1
  [VTQD_VehActSpd_kph] -> Relational Operator2/1
  Constant14/1 -> Relational Operator2/2
  [VTQD_GearActualPosn_enum] -> Equal9/1
  Constant11/1 -> Equal9/2
  [VTQD_GearActualPosn_enum] -> Delay2/1
  [task_time_s] -> DelayEnable/3
  [VVMC_EstSlope_Deg] -> Relational Operator1/1
  DelayEnable/1 -> SR_Latch4/2  "VTQD_R2DEnOPDHold_flg"
  Constant13/1 -> Relational Operator1/2
  [VTQD_OPDHoldR2D_flg] -> Delay3/1
  Constant12/1 -> Relational Operator/2
  Delay2/1 -> Equal6/1
  OR/1 -> SR_Latch3/2
  Delay/1 -> OR/1
  Equal5/1 -> AND/2
  [VTQD_RegenMode_enum] -> Equal4/1
  AND/1 -> OR/2
  Constant8/1 -> Equal4/2
  [VTQD_GearActualPosn_enum] -> Equal5/1
  Equal4/1 -> AND/1
  Constant9/1 -> Equal5/2
  [VTQD_OPDHoldRgnOn2Off_flg] -> VTQD_OPDHoldRgnOn2Off_flg/1
  [VTQD_OPDHoldDelayForP_flg] -> VTQD_OPDHoldDelayForP_flg/1
  [VTQD_APSStaSys_enum] -> VTQD_APSStaSys_enum/1
  VTQD_VehActSpd_kph/1 -> [VTQD_VehActSpd_kph]
  VVMC_CruzActive_flg/1 -> [VVMC_CruzActive_flg]
  VPMM_PwrSta_enum/1 -> [VPMM_PwrSta_enum]
  VVMC_ADASActive_flg/1 -> [VVMC_ADASActive_flg]
  VTQD_AutiHoldRelease_flg/1 -> [VTQD_AutiHoldRelease_flg]
  VTQD_RegenMode_enum/1 -> [VTQD_RegenMode_enum]
  VINP_EPBSta_enum/1 -> [VINP_EPBSta_enum]
  VTQD_GearActualPosn_enum/1 -> [VTQD_GearActualPosn_enum]
  Constant4/1 -> Equal1/2
  [VINP_EPBSta_enum] -> Equal10/1
  Constant3/1 -> Equal10/2
  [VTQD_RegenMode_enum] -> Equal11/1
  Constant44/1 -> Equal11/2
  [VTQD_AutiHoldRelease_flg] -> Delay/1
  Unit Delay1/1 -> GreaterThan3/1
  Equal30/1 -> AND6/1
  [VPMM_PwrSta_enum] -> Equal30/1
  AND6/1 -> SR_Latch3/1
  Constant45/1 -> Equal30/2
  GreaterThan3/1 -> AND6/2
  SR_Latch3/1 -> [VTQD_OPDHoldRgnOn2Off_flg]  "VTQD_OPDHoldRgnOn2Off_flg"
  Equal11/1 -> Unit Delay1/1, GreaterThan3/2
  Equal10/1 -> AND5/2
  AND5/1 -> [VTQD_OPDHoldDelayForP_flg]  "VTQD_OPDHoldDelayForP_flg"
  Equal1/1 -> AND5/1
  [VTQD_GearActualPosn_enum] -> Equal1/1
  Constant1/1 -> Switch/1
  Constant2/1 -> Switch/3
  Switch/1 -> [VTQD_APSStaSys_enum]  "VTQD_APSStaSys_enum"
  AND2/1 -> OR4/1
  [VTQD_OPDHoldForceEn_flg] -> OR4/2
  OR4/1 -> Switch/2
  Abs/1 -> Switch1/1
  [VTQD_TqTargetShaftSpd_rpm] -> Abs/1
  Equal19/1 -> Detect Increase/1
  Detect Increase/1 -> Switch1/2
  [VTQD_ForceOPDHoldEnDelay_s] -> DelayEnable2/2
  Constant26/1 -> Equal17/2
  [VINP_DrDoorSW_flg] -> AND12/2
  Equal12/1 -> AND12/1
  Constant24/1 -> Equal12/2
  [VTQD_GearActualPosn_enum] -> Equal12/1
  [VTQD_BrkSwSta_flg] -> AND11/2
  Add/1 -> Relational Operator6/1
  Constant25/1 -> Equal16/2
  OR2/1 -> SR_Latch1/2, SR_Latch2/2
  AND10/1 -> Switch3/1
  [VTQD_GearActualPosn_enum] -> Equal19/1
  [VINP_MCPressure_bar] -> MTQD_AccIneOPDHoldEnDelay_Z_s/1
  [VTQD_TqTargetShaftSpd_rpm] -> Add/1
  Detect Change/1 -> AND11/1
  Equal18/1 -> OR2/2
  SR_Latch2/1 -> [VTQD_OPDHoldForceEn_flg]  "VTQD_OPDHoldForceEn_flg"
  [VINP_EPBSta_enum] -> Equal16/1
  MTQD_DecIneOPDHoldEnDelay_Z_s/1 -> Switch2/3  "VTQD_DecIneOPDHoldEnDelay_s"
  MTQD_AccIneOPDHoldEnDelay_Z_s/1 -> Switch2/1  "VTQD_AccIneOPDHoldEnDelay_s"
  Switch1/1 -> Add/2, Delay1/1  "VTQD_OPDHoldMemShaftSpd_rpm"
  Constant29/1 -> Relational Operator6/2
  [VTQD_ForceP_flg] -> AND10/1
  AND11/1 -> OR2/3
  Constant31/1 -> Switch3/2
  Relational Operator6/1 -> Switch2/2  "VTQD_InertialDirection_flg"
  [VVMC_EstSlope_Deg] -> MTQD_DecIneOPDHoldEnDelay_Z_s/2
  [VTQD_EPBCarWashMode_flg] -> OR2/1
  Switch3/1 -> SR_Latch1/1
  [VVMC_EstSlope_Deg] -> MTQD_AccIneOPDHoldEnDelay_Z_s/2
  Equal20/1 -> AND10/2
  [VINP_DriverSeatBeltCmd_flg] -> OR6/2
  Equal16/1 -> AND12/4
  DelayEnable2/1 -> SR_Latch2/1
  Constant27/1 -> Equal18/2
  Switch2/1 -> [VTQD_ForceOPDHoldEnDelay_s]  "VTQD_ForceOPDHoldEnDelay_s"
  [VINP_EPBSta_enum] -> Equal20/1
  Delay1/1 -> Switch1/3
  [VINP_ShifterHandleCmd_enum] -> Detect Change/1
  [VINP_EPBSta_enum] -> Equal18/1
  [VINP_MCPressure_bar] -> MTQD_DecIneOPDHoldEnDelay_Z_s/1
  Constant28/1 -> Equal19/2
  [task_time_s] -> DelayEnable2/3
  OR6/1 -> AND12/3
  Equal17/1 -> OR6/1
  Constant30/1 -> Equal20/2
  AND12/1 -> Switch3/3
  SR_Latch1/1 -> DelayEnable2/1
  [VPMM_DrSeatSta_enum] -> Equal17/1
  VTQD_ForceP_flg/1 -> [VTQD_ForceP_flg]
  VINP_DrDoorSW_flg/1 -> [VINP_DrDoorSW_flg]
  VPMM_DrSeatSta_enum/1 -> [VPMM_DrSeatSta_enum]
  VTQD_EPBCarWashMode_flg/1 -> [VTQD_EPBCarWashMode_flg]
  VINP_ShifterHandleCmd_enum/1 -> [VINP_ShifterHandleCmd_enum]
  VTQD_BrkSwSta_flg/1 -> [VTQD_BrkSwSta_flg]
  VTQD_TqTargetShaftSpd_rpm/1 -> [VTQD_TqTargetShaftSpd_rpm]
  VINP_DriverSeatBeltCmd_flg/1 -> [VINP_DriverSeatBeltCmd_flg]
  VINP_MCPressure_bar/1 -> [VINP_MCPressure_bar]
  [VTQD_OPDHoldForceEn_flg] -> VTQD_OPDHoldForceEn_flg/1

== system tqdtqr_rebuild_V3/Input_Convert/Signal function/Regen level define/OUTPUT ONLY ON or READY ==
  note: INPUT Signals
  VPMM_PowerSta_enum : Inport
  VTQD_SWCRegenUpSta_flg : Inport  Port=2
  VTQD_SWCRegenDownSta_flg : Inport  Port=3
  VINP_ADASACCSta_enum : Inport  Port=4
  VVMC_CCCtrlSta_enum : Inport  Port=5
  VBCM_BrakeLamp_flg : Inport  Port=6
  VINP_VehSpeed_kph : Inport  Port=7
  AND : Logic  Inputs=6  AllPortsSameDT=off  OutDataTypeStr=boolean
  Constant1 : Constant  Value=ENUM_ADASACCSTA_ACTIVE
  Constant10 : Constant  Value=FALSE
  Constant11 : Constant  Value=KTQD_RegenButEnSpd_kph
  Constant3 : Constant  Value=ENUM_POWERSTA_ON
  Constant5 : Constant  Value=FALSE
  Constant6 : Constant  Value=ENUM_ADASACCSTA_OVERRIDE
  Constant7 : Constant  Value=ENUM_POWERSTA_READY
  Constant8 : Constant  Value=ENUM_ADASCCSTA_ACTIVE
  Constant9 : Constant  Value=ENUM_ADASCCSTA_OVRRIDE
  Equal2 : RelationalOperator  Operator===  OutDataTypeStr=boolean  RndMeth=Simplest
  Equal3 : RelationalOperator  Operator===  OutDataTypeStr=boolean  RndMeth=Simplest
  Equal{4..7} (4 alike) : RelationalOperator  Operator=~=  OutDataTypeStr=boolean  RndMeth=Simplest
  NOT : Logic  Operator=NOT  AllPortsSameDT=off  OutDataTypeStr=boolean
  OR1 : Logic  Operator=OR  AllPortsSameDT=off  OutDataTypeStr=boolean
  OR2 : Logic  Operator=OR  AllPortsSameDT=off  OutDataTypeStr=boolean
  Relational Operator : RelationalOperator  Operator=<=  OutDataTypeStr=boolean  RndMeth=Simplest
  Switch : Switch  Criteria=u2 ~= 0
      settings: AttributesFormatString=%<Criteria>
  Switch1 : Switch  Criteria=u2 ~= 0
      settings: AttributesFormatString=%<Criteria>
  SWC_RegenUp : Outport
  SWC_RegenDown : Outport  Port=2
  wires:
  [VPMM_PowerSta_enum] -> Equal3/1
  Equal2/1 -> OR1/1
  Constant3/1 -> Equal2/2
  Constant7/1 -> Equal3/2
  [VPMM_PowerSta_enum] -> Equal2/1
  Equal3/1 -> OR1/2
  [VINP_ADASACCSta_enum] -> Equal4/1
  Constant1/1 -> Equal4/2
  Constant6/1 -> Equal5/2
  [VINP_ADASACCSta_enum] -> Equal5/1
  [VVMC_CCCtrlSta_enum] -> Equal6/1
  [VVMC_CCCtrlSta_enum] -> Equal7/1
  [VBCM_BrakeLamp_flg] -> NOT/1
  Constant9/1 -> Equal7/2
  Constant8/1 -> Equal6/2
  OR1/1 -> AND/1
  Equal7/1 -> AND/5
  Equal6/1 -> AND/4
  Equal5/1 -> AND/3
  Equal4/1 -> AND/2
  [VINP_VehSpeed_kph] -> Relational Operator/1
  Constant11/1 -> Relational Operator/2
  OR2/1 -> AND/6
  NOT/1 -> OR2/1
  Relational Operator/1 -> OR2/2
  VINP_VehSpeed_kph/1 -> [VINP_VehSpeed_kph]
  VBCM_BrakeLamp_flg/1 -> [VBCM_BrakeLamp_flg]
  VVMC_CCCtrlSta_enum/1 -> [VVMC_CCCtrlSta_enum]
  VINP_ADASACCSta_enum/1 -> [VINP_ADASACCSta_enum]
  VPMM_PowerSta_enum/1 -> [VPMM_PowerSta_enum]
  AND/1 -> Switch/2, Switch1/2
  Constant10/1 -> Switch1/3
  Switch1/1 -> SWC_RegenDown/1  "SWC_RegenDown"
  VTQD_SWCRegenDownSta_flg/1 -> Switch1/1
  VTQD_SWCRegenUpSta_flg/1 -> Switch/1
  Switch/1 -> SWC_RegenUp/1  "SWC_RegenUp"
  Constant5/1 -> Switch/3

== system tqdtqr_rebuild_V3/Input_Convert/Signal function/Regen level define/Regen Level Switch Botton ==
  task_time_s : Inport
  SWC_RegenUp : Inport  Port=2
  SWC_RegenDown : Inport  Port=3
  VINP_DIDNVHPedalLim_flg : Inport  Port=4
  Constant1 : Constant  Value=ENUM_REGENSWSTA_NOACTION
  Constant13 : Constant  Value=ENUM_REGENSWSTA_SHORTPRESSUP
  Constant18 : Constant  Value=ENUM_REGENSWSTA_LONGPRESSUP
  Constant21 : Constant  Value=ENUM_REGENSWSTA_SHORTPRESSDOWN
  Constant23 : Constant  Value=ENUM_REGENSWSTA_LONGPRESSDOWN
  Constant24 : Constant  Value=ENUM_REGENSWSTA_NOACTION
  RegenDOWN : Subsystem
  RegenUP : Subsystem
  Switch{1,4,6..8} (5 alike) : Switch  Criteria=u2 ~= 0
      Switch4 settings: AttributesFormatString=%<Criteria>
      Switch6 settings: AttributesFormatString=%<Criteria>
      Switch7 settings: AttributesFormatString=%<Criteria>
      Switch8 settings: AttributesFormatString=%<Criteria>
  VTQD_RegenSWSta_enum : Outport
  wires:
  [task_time_s] -> RegenDOWN/1(task_time_s)
  [task_time_s] -> RegenUP/1(task_time_s)
  task_time_s/1 -> [task_time_s]
  Switch8/1 -> Switch7/3
  SWC_RegenDown/1 -> [SWC_RegenDown]
  SWC_RegenUp/1 -> [SWC_RegenUP]
  [SWC_RegenDown] -> RegenUP/3(SWC_RegenDOWN)
  RegenUP/1(SWC_RegenUpShort_flg) -> Switch4/2
  Switch6/1 -> Switch4/3
  RegenUP/2(VTQD_RegenUpLongP_flg) -> Switch6/2
  Constant18/1 -> Switch6/1
  [SWC_RegenUP] -> RegenDOWN/2(SWC_RegenUp)
  RegenDOWN/1(SWC_RegenDownShort_flg) -> Switch7/2
  Switch7/1 -> Switch6/3
  Constant21/1 -> Switch7/1
  Constant23/1 -> Switch8/1
  RegenDOWN/2(VTQD_RegenDownLongP_flg) -> Switch8/2
  [SWC_RegenDown] -> RegenDOWN/3(SWC_RegenDOWN)
  Constant13/1 -> Switch4/1
  Constant24/1 -> Switch8/3
  [SWC_RegenUP] -> RegenUP/2(SWC_RegenUp)
  VINP_DIDNVHPedalLim_flg/1 -> [VINP_DIDNVHPedalLim_flg]
  Switch1/1 -> VTQD_RegenSWSta_enum/1
  Constant1/1 -> Switch1/1
  [VINP_DIDNVHPedalLim_flg] -> Switch1/2
  Switch4/1 -> Switch1/3
